simulink model "sl_jointspace"  (R2022b)
settings: Solver=VariableStepDiscrete  StartTime=0.0  StopTime=2  MaxStep=0.02  RelTol=1e-3
PreLoadFcn:
  | % Load ABB robot, so it's available for forward kinematics
  | abb = loadrobot("abbIrb1600", DataFormat="row");
libraries: robotcorelib x2, robotmaniplib x1
settings Model: Creator=rpill  LastModifiedBy=rpillat
settings SolverCC: MaxZcPerStep=1
settings ModelReferenceCC: EnableRefExpFcnMdlSchedulingChecks=on
settings RTWCC: DLArmComputeVersion=19.05

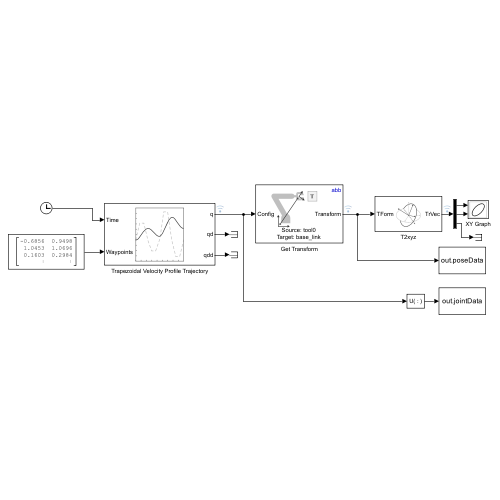
[thumbnail: Simulink's stored preview of the top-level diagram]
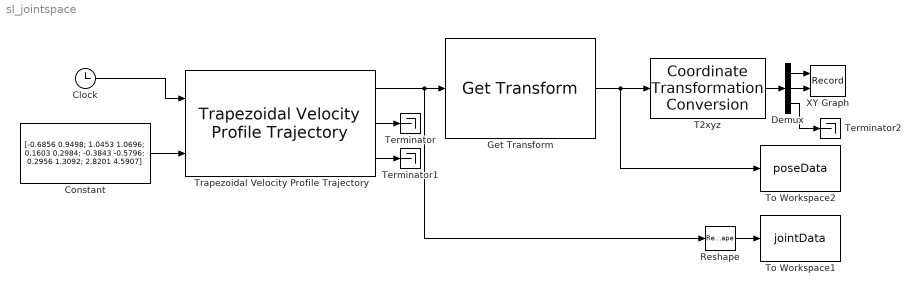
== system sl_jointspace ==
  Clock : Clock
  Constant : Constant  Value=[-0.6856 0.9498; 1.0453 1.0696; 0.1603 0.2984; -0.3843 -0.5796; 0.2956 1.3092; 2.8201 4.5907]
  Demux : Demux  Outputs=3
  Get Transform : robotmaniplib/Get Transform  RigidBodyTree=abb  SourceBody=tool0  TargetBody=base_link  SimulateUsing=Interpreted execution
  Reshape : Reshape
  T2xyz : robotcorelib/Coordinate Transformation Conversion  InputRepresentation=Homogeneous Transformation  InputEulerSequence=ZYX  ShowTrVecInputPort=on  OutputRepresentation=Translation Vector  OutputEulerSequence=ZYX  ShowTrVecOutputPort=on  SimulateUsing=Interpreted execution
  Terminator : Terminator
  Terminator1 : Terminator
  Terminator2 : Terminator
  To Workspace1 : ToWorkspace  VariableName=jointData  SampleTime=-1
      settings: Save2DSignal=2-D array (concatenate along first dimension)
  To Workspace2 : ToWorkspace  VariableName=poseData  SampleTime=-1
  Trapezoidal Velocity Profile Trajectory : robotcorelib/Trapezoidal Velocity Profile Trajectory  WaypointSource=External  Waypoints=[ 0, -0.5, -1; 0, 0.5, 1 ]  NumParams=1  Parameter1=End Time  Parameter2=End Time  ParameterSource=Internal  PeakVelocity=[ 2; 2 ]  Acceleration=[ 1; 2 ]  EndTime=2  AccelTime=[ 1; 2 ]  SimulateUsing=Interpreted execution
  XY Graph : Record  FileSettingsInternal="{\"entries\":[{\"content\":{\"excelSettings\":{\"content\":{},\"type\":\"Streamout.ExcelSettings\"}},\"type\":\"Streamout.FileSettingStorage\",\"uuid\":\"86787838-974e-41be-9360-27d0aee75d48\"}],\"packageUris\":[\"http://schema.mathworks.com/mf0/streamout_blocks/R2020a\"],\"version\":\"1.0\"}"  Layout=[1 1]  SignalsInternal="{\"entries\":[{\"content\":{\"signals\":[{\"content\":{\"blockPath\":[\"sl_jointspace_22b/XY Graph\"],\"channel\":[],\"dimensions\":[1,1],\"domain\":\"sl_jointspace_22b/XY Graph\",\"lineColor\":\"#a2142f\",\"plots\":[1],\"port\":1,\"sid\":[],\"signalID\":584,\"signalName\":\"Demux:1\"},\"type\":\"RecordBlkView.Signal\",\"uuid\":\"8a11348d-2b9a-4abc-9d96-94ce55a1e1f6\"},{\"content\":{\"blockPath\":[\"sl_jointspace_22b/XY Graph\"],\"channel\":[],\"dimensions\":[1,1],\"domain\":\"sl_jointspace_22b/XY Graph\",\"lineColor\":\"#139fff\",\"plots\":[1],\"port\":2,\"sid\":[],\"signalID\":587,\"signalName\":\"Demux:2\"},\"type\":\"RecordBlkView.Signal\",\"uuid\":\"b38ac7e4-1e37-4849-92cf-8d203b0952b5\"}]},\"type\":\"RecordBlkView.InputSignals\",\"uuid\":\"4bb1be58-cfcc-440c-b07b-cda6993e2993\"}],\"packageUris\":[\"http://schema.mathworks.com/mf0/streamout_blocks/R2020a\"],\"version\":\"1.0\"}"  VisualizationBindings="{\"xyplotplugin\":{\"info\":[{\"series\":[{\"bindingParametersList\":[{\"parameter\":\"X-Axis\",\"signalID\":584,\"signalName\":\"Demux:1\"},{\"parameter\":\"Y-Axis\",\"signalID\":587,\"signalName\":\"Demux:2\"}],\"seriesID\":52801}],\"subplotID\":1}]}}"  CompatibilityTag=XY
  wires:
  Constant/1 -> Trapezoidal Velocity Profile Trajectory/2
  Clock/1 -> Trapezoidal Velocity Profile Trajectory/1
  Trapezoidal Velocity Profile Trajectory/2 -> Terminator/1
  Trapezoidal Velocity Profile Trajectory/3 -> Terminator1/1
  Trapezoidal Velocity Profile Trajectory/1 -> Reshape/1, Get Transform/1
  Get Transform/1 -> To Workspace2/1, T2xyz/1
  T2xyz/1 -> Demux/1
  Demux/2 -> XY Graph/2
  Demux/1 -> XY Graph/1
  Reshape/1 -> To Workspace1/1
  Demux/3 -> Terminator2/1
